simulink model "simplePendulem"  (R2017a)
settings: Solver=ode45  StartTime=0.0  StopTime=20.0  RelTol=1e-3  EnableMultiTasking=on
settings Model: Creator=edward  LastModifiedBy=edward
settings DataIOCC: LimitDataPoints=on  SaveFormat=Array
settings OptimizationCC: LifeSpan=inf
settings DebuggingCC: UnderspecifiedInitializationDetection=Classic  MergeDetectMultiDrivingBlocksExec=none  SolverPrmCheckMsg=warning  SFUnexpectedBacktrackingDiag=warning  SFNoUnconditionalDefaultTransitionDiag=warning  SFExecutionAtInitializationDiag=none
settings HardwareCC: ProdBitPerPointer=32  ProdBitPerSizeT=32  ProdBitPerPtrDiffT=32  ProdLargestAtomicFloat=None  ProdIntDivRoundTo=Undefined  ProdEndianess=Unspecified  ProdWordSize=32  ProdHWDeviceType=32-bit Generic
settings ModelReferenceCC: PropagateSignalLabelsOutOfModel=off
settings GRTTargetCC: TargetLangStandard=C89/C90 (ANSI)  GeneratePreprocessorConditionals=Disable all
settings ConfigComp: CovMetricSettings=dw  CovHtmlReporting=on  CovSaveCumulativeToWorkspaceVar=on  CovSaveSingleToWorkspaceVar=on  CovExternalEMLEnable=off

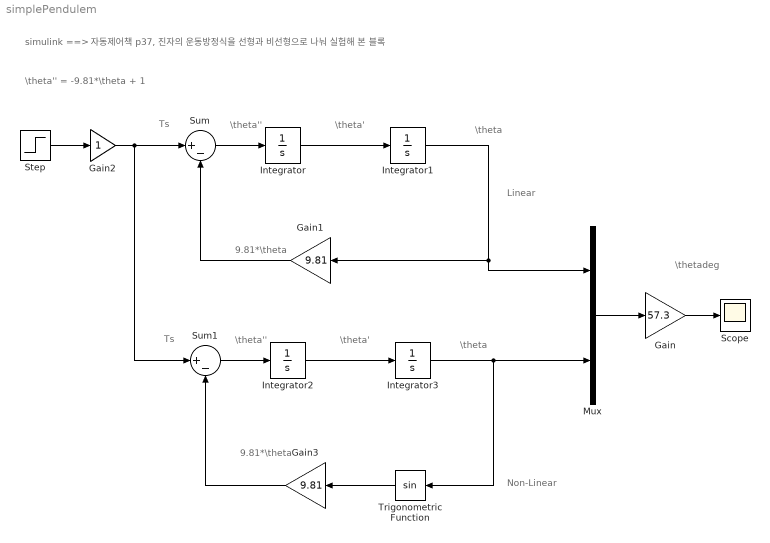
== system simplePendulem ==
  note: \theta'' = -9.81*\theta + 1
  note: simulink ==> 자동제어책 p37, 진자의 운동방정식을 선형과 비선형으로 나눠 실험해 본 블록
  note: Non-Linear
  note: \theta''
  note: Ts
  note: \theta'
  note: \theta
  note: 9.81*\theta
  note: \thetadeg
  note: \theta''
  note: Ts
  note: \theta'
  note: \theta
  note: 9.81*\theta
  note: Linear
  Gain : Gain  Gain=57.3
  Gain1 : Gain  Gain=9.81
  Gain2 : Gain
  Gain3 : Gain  Gain=9.81
  Integrator{,1..3} (4 alike) : Integrator
  Mux : Mux  Inputs=2
  Scope : Scope
  Step : Step  SampleTime=0
  Sum : Sum  Inputs=|+-
  Sum1 : Sum  Inputs=|+-
  Trigonometric Function : Trigonometry
  wires:
  Step/1 -> Gain2/1
  Sum/1 -> Integrator/1
  Integrator/1 -> Integrator1/1
  Integrator1/1 -> Mux/1, Gain1/1
  Gain1/1 -> Sum/2
  Gain/1 -> Scope/1
  Mux/1 -> Gain/1
  Sum1/1 -> Integrator2/1
  Integrator2/1 -> Integrator3/1
  Integrator3/1 -> Trigonometric Function/1, Mux/2
  Gain3/1 -> Sum1/2
  Gain2/1 -> Sum/1, Sum1/1
  Trigonometric Function/1 -> Gain3/1
